simulink model "controls_pert_saida"  (R2022a)
settings: Solver=FixedStepDiscrete  StartTime=0.0  StopTime=30  FixedStep=dt  RelTol=1e-3
undefined symbols (not defined in the file or in its folder): R_z2, S_z2, T_z2
libraries: cstblocks x1
settings Model: Creator=phcs  LastModifiedBy=phcs

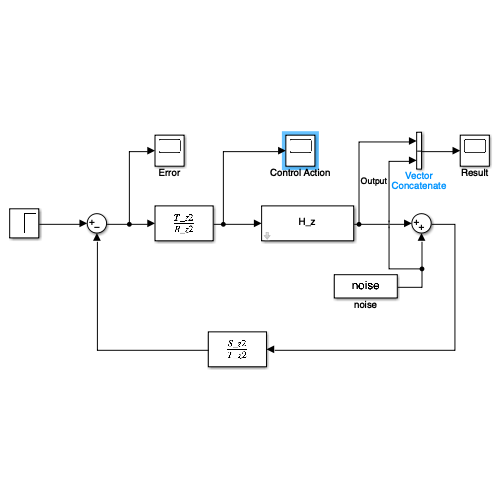
[thumbnail: Simulink's stored preview of the top-level diagram]
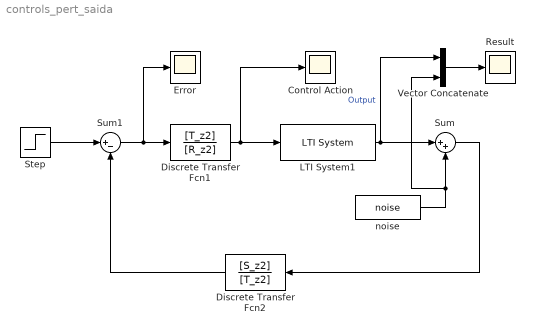
== system controls_pert_saida ==
  Control Action : Scope
  Discrete Transfer Fcn1 : DiscreteTransferFcn  Numerator=[T_z2]  Denominator=[R_z2]
  Discrete Transfer Fcn2 : DiscreteTransferFcn  Numerator=[S_z2]  Denominator=[T_z2]
  Error : Scope
  LTI System1 : cstblocks/LTI System  sys=H_z  IC=[]
  Result : Scope
  Step : Step  Time=0  After=0  SampleTime=0
  Sum : Sum  Inputs=|++
  Sum1 : Sum  Inputs=|+-
  Vector Concatenate : Concatenate
  noise : FromWorkspace  VariableName=noise
  wires:
  Discrete Transfer Fcn2/1 -> Sum1/2
  Discrete Transfer Fcn1/1 -> LTI System1/1, Control Action/1
  Step/1 -> Sum1/1
  Sum1/1 -> Error/1, Discrete Transfer Fcn1/1
  LTI System1/1 -> Vector Concatenate/1, Sum/1  "Output"
  Sum/1 -> Discrete Transfer Fcn2/1
  noise/1 -> Vector Concatenate/2, Sum/2
  Vector Concatenate/1 -> Result/1
